simulink model "untitled"  (R2021a)
settings: Solver=VariableStepAuto  StartTime=0.0  StopTime=10.0  RelTol=1e-3
libraries: dspxfrm3 x3, dspmtrx3 x2, dspbuff3 x1, dspsigops x1
settings Model: Creator=Kimo Store  LastModifiedBy=Kimo Store

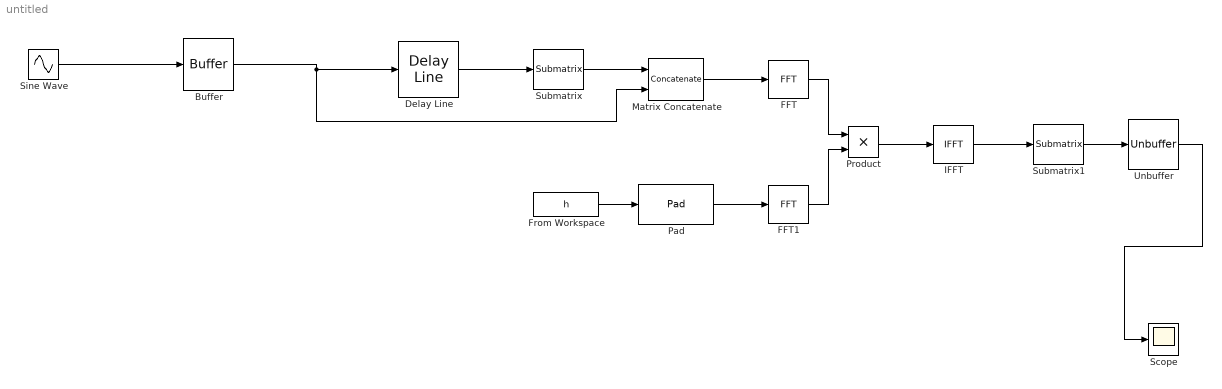
== system untitled ==
  Buffer : Buffer  N=400  OutputFrames=off
  Delay Line : dspbuff3/Delay Line  siz=400  ic=0  directfeed=off  enable_output=off  hold_output=off  OutputFrames=off
      settings: SourceProductBaseCode=DS
  FFT : dspxfrm3/FFT  FFTImplementation=Auto  CompMethod=Table lookup  TableOpt=NEW  TableOptActive=Speed  BitRevOrder=off  Normalize=off  InheritFFTLength=on  FFTLength=64  WrapInput=on  roundingMode=Floor  overflowMode=off  firstCoeffDataTypeStr=Inherit: Same word length as input  firstCoeffLastDataTypeStr=Inherit: Same word length as input  outputMin=[]  outputMax=[]
  FFT1 : dspxfrm3/FFT  FFTImplementation=Auto  CompMethod=Table lookup  TableOpt=NEW  TableOptActive=Speed  BitRevOrder=off  Normalize=off  InheritFFTLength=on  FFTLength=64  WrapInput=on  roundingMode=Floor  overflowMode=off  firstCoeffDataTypeStr=Inherit: Same word length as input  firstCoeffLastDataTypeStr=Inherit: Same word length as input  outputMin=[]  outputMax=[]
  From Workspace : FromWorkspace  VariableName=h  SampleTime=400/8000
  IFFT : dspxfrm3/IFFT  FFTImplementation=Auto  CompMethod=Table lookup  TableOpt=NEW  TableOptActive=Speed  BitRevOrder=off  cs_in=on  Normalize=on  InheritFFTLength=on  FFTLength=64  WrapInput=on  mode=Complex  outSamplingMode=Sample based  roundingMode=Floor  overflowMode=off  firstCoeffDataTypeStr=Inherit: Same word length as input  firstCoeffLastDataTypeStr=Inherit: Same word length as input  outputMin=[]  outputMax=[]
  Matrix Concatenate : Concatenate  Mode=Multidimensional array
  Pad : dspsigops/Pad  padAlong=Columns  dimsToPad=1  valSrc=Specify via dialog  padVal=0  spec=Output size  padNumOutRowsSpecMethod=User-specified  numOutRows=512  padNumOutColsSpecMethod=User-specified  numOutCols=1  isVarDimsMode=off  padBeginning=0  padEnd=0  outSizeMode=User-specified  outSize=1  padSigAt=End  trunc_flag=None  roundingMode=Floor  overflowMode=off  truncOrWrapMode=Truncate  wrap_flag=None
      settings: SourceProductBaseCode=DS
  Product : Product
  Scope : Scope
  Sine Wave : Sin  Frequency=100  SampleTime=1/8000
  Submatrix : dspmtrx3/Submatrix  RowSpan=Range of rows  RowStartMode=Index  RowStartIndex=289  RowEndMode=Last  RowEndIndex=1  ColSpan=All columns  ColStartMode=First  ColStartIndex=1  ColEndMode=Last  ColEndIndex=1
  Submatrix1 : dspmtrx3/Submatrix  RowSpan=Range of rows  RowStartMode=Index  RowStartIndex=113  RowEndMode=Last  RowEndIndex=1  ColSpan=All columns  ColStartMode=First  ColStartIndex=1  ColEndMode=Last  ColEndIndex=1
  Unbuffer : Unbuffer
  wires:
  Delay Line/1 -> Submatrix/1
  Submatrix/1 -> Matrix Concatenate/1
  Buffer/1 -> Delay Line/1, Matrix Concatenate/2
  Matrix Concatenate/1 -> FFT/1
  From Workspace/1 -> Pad/1
  Pad/1 -> FFT1/1
  FFT/1 -> Product/1
  FFT1/1 -> Product/2
  Product/1 -> IFFT/1
  IFFT/1 -> Submatrix1/1
  Submatrix1/1 -> Unbuffer/1
  Unbuffer/1 -> Scope/1
  Sine Wave/1 -> Buffer/1
